simulink model "val_discrete_model"  (R2026a)
settings: Solver=VariableStepAuto  StopTime=1000
undefined symbols (not defined in the file): filter_param, plant_param, r_param
libraries: lib_plant x1
settings Model: Creator=alessandro-nardin  LastModifiedBy=alessandro-nardin

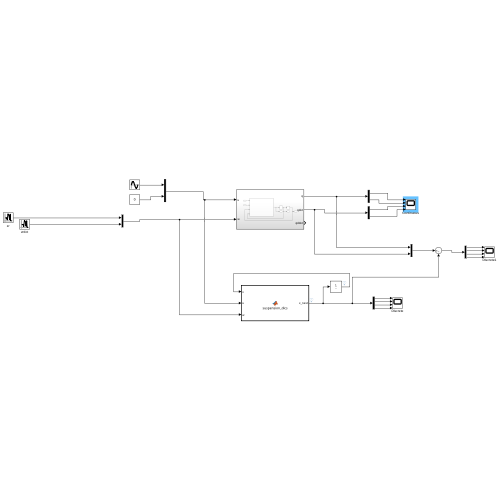
[thumbnail: Simulink's stored preview of the top-level diagram]
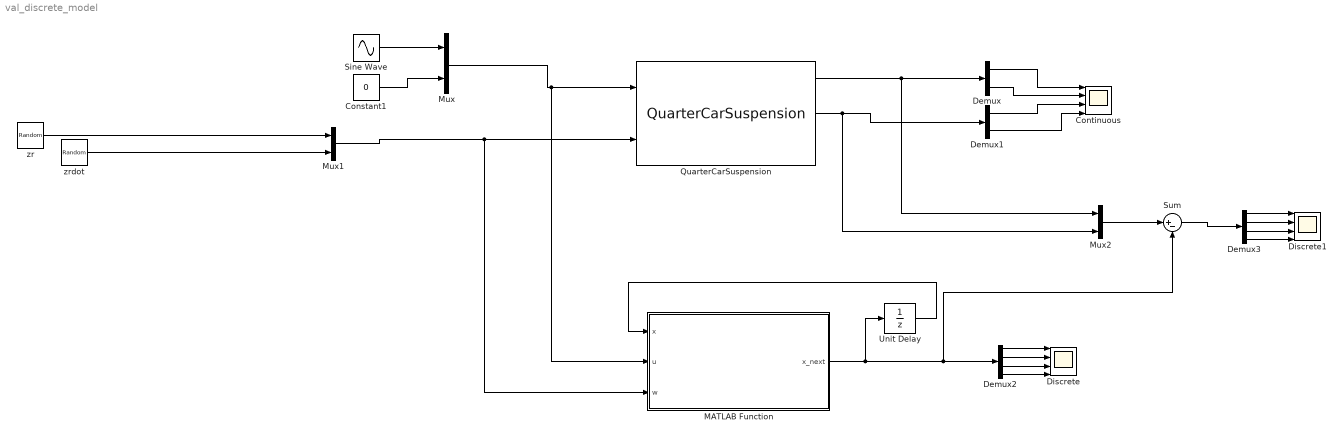
== system val_discrete_model ==
  Constant1 : Constant  Value=0
  Continuous : Scope  NumInputPorts=4
      settings: ActiveDisplayYMinimum=-16.159253363263144  ActiveDisplayYMaximum=16.375252619446012
  Demux : Demux  Outputs=2
  Demux1 : Demux  Outputs=2
  Demux2 : Demux
  Demux3 : Demux
  Discrete : Scope  NumInputPorts=4
      settings: ActiveDisplayYMinimum=-16.176369892438977  ActiveDisplayYMaximum=16.393597358066664
  Discrete1 : Scope  NumInputPorts=4
      settings: ActiveDisplayYMinimum=-0.190499153731658  ActiveDisplayYMaximum=0.17591013542810041  DataLoggingVariableName=ScopeData2
  MATLAB Function : MATLAB Function  TreatAsAtomicUnit=on
  Mux : Mux  Inputs=2
  Mux1 : Mux  Inputs=2
  Mux2 : Mux  Inputs=2
  QuarterCarSuspension : lib_plant/QuarterCarSuspension  SystemSampleTime=-1  VariantActivationTime=update diagram  EmptyChoice=off  PassThrough=off  PassThroughVariantControl=(default)  EmptyChoiceVariantControl=(default)  AllowFlexibleInterface=on  Latency=0  AutoFrameSizeCalculation=off
      settings: SourceProductName=Lib Plant
  Sine Wave : Sin  Amplitude=1000  Frequency=0.5  SampleTime=0
  Sum : Sum  Inputs=|+-
  Unit Delay : UnitDelay  SampleTime=-1
  zr : RandomNumber  Variance=r_param.rz_var  SampleTime=0.1
  zrdot : RandomNumber  Variance=r_param.rzdot_var  Seed=1  SampleTime=0.1
  wires:
  MATLAB Function/1(x_next) -> Unit Delay/1, Sum/2, Demux2/1
  Mux1/1 -> MATLAB Function/3(w), QuarterCarSuspension/2
  Sine Wave/1 -> Mux/1
  Constant1/1 -> Mux/2
  Mux/1 -> MATLAB Function/2(u), QuarterCarSuspension/1
  QuarterCarSuspension/1 -> Mux2/1, Demux/1
  QuarterCarSuspension/2 -> Mux2/2, Demux1/1
  Demux2/4 -> Discrete/4
  Demux2/3 -> Discrete/3
  Demux2/1 -> Discrete/1
  Demux2/2 -> Discrete/2
  Demux/1 -> Continuous/1
  Demux/2 -> Continuous/2
  Demux1/1 -> Continuous/3
  Demux1/2 -> Continuous/4
  Unit Delay/1 -> MATLAB Function/1(x)
  zr/1 -> Mux1/1
  zrdot/1 -> Mux1/2
  Mux2/1 -> Sum/1
  Sum/1 -> Demux3/1
  Demux3/4 -> Discrete1/4
  Demux3/3 -> Discrete1/3
  Demux3/1 -> Discrete1/1
  Demux3/2 -> Discrete1/2

== matlab function val_discrete_model/MATLAB Function ==
  settings: updateMethod=DISCRETE  sampleTime=filter_param.sample_t
  data: x input; u input; x_next output size=[ 4 1 ]; w input; plant_param parameter; filter_param parameter
function x_next = suspension_dics( x, u, w, plant_param, filter_param)
x_next = suspension_f_dics_euler( x, u, w, plant_param, filter_param.sample_t);
